simulink model "stab_full_loop"  (R2021a)
settings: Solver=VariableStepAuto  StartTime=0.0  StopTime=5  RelTol=1e-3
values from neighbouring files (symbols this model uses):
  Ahs3 = blkdiag(Ahs3, Ahcs)    [ranger_full_indi_sim.m]
  Ahs7 = blkdiag(Ahs7, Ahcs)    [ranger_full_indi_sim.m]
  Amc = d2c(Amd,'tustin')    [ranger_full_indi_sim.m]
  Asc = d2c(Asd,'tustin')    [ranger_full_indi_sim.m]
  Bhs3 = blkdiag(Bhs3, Bhcs)    [ranger_full_indi_sim.m]
  Bhs7 = blkdiag(Bhs7, Bhcs)    [ranger_full_indi_sim.m]
  Chs3 = blkdiag(Chs3, Chcs)    [ranger_full_indi_sim.m]
  Chs7 = blkdiag(Chs7, Chcs)    [ranger_full_indi_sim.m]
  Dhs3 = blkdiag(Dhs3, Dhcs)    [ranger_full_indi_sim.m]
  Dhs7 = blkdiag(Dhs7, Dhcs)    [ranger_full_indi_sim.m]
  Gs = [-10.67  10.67  0     0     0     0 0 ... (first row only)    [ranger_full_indi_sim.m]
  Gs_inv = pinv(Gs)    [ranger_full_indi_sim.m]
  Gs_thrust = [0 0 0 0 0 0 0 ... (first row only)    [ranger_full_indi_sim.m]
  Kds = [10; 18; 18]    [ranger_full_indi_sim.m]
  Kps = [4.1089; 4.7304; 7.36]    [ranger_full_indi_sim.m]
settings Model: Creator=AutomZ2-RG02B04  LastModifiedBy=AutomZ2-RG02A02
settings SolverCC: AlgebraicLoopSolver=TrustRegion

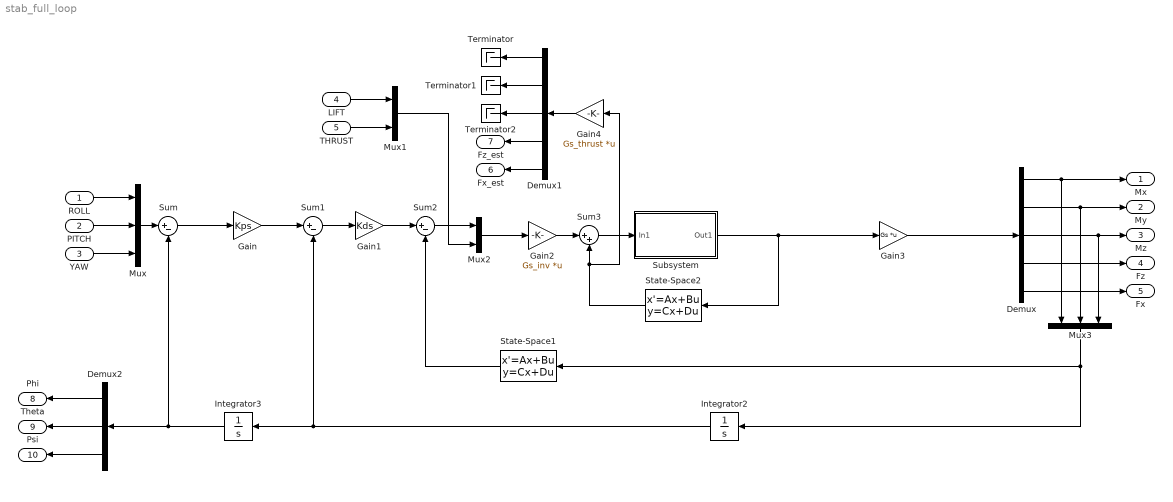
== system stab_full_loop ==
  ROLL : Inport
  PITCH : Inport  Port=2
  YAW : Inport  Port=3
  LIFT : Inport  Port=4
  THRUST : Inport  Port=5
  Demux : Demux  Outputs=5
  Demux1 : Demux  Outputs=5
  Demux2 : Demux  Outputs=3
  Gain : Gain  Gain=Kps
  Gain1 : Gain  Gain=Kds
  Gain2 : Gain  Gain=Gs_inv  Multiplication=Matrix(K*u)
  Gain3 : Gain  Gain=Gs  Multiplication=Matrix(K*u)
  Gain4 : Gain  Gain=Gs_thrust  Multiplication=Matrix(K*u)
  Integrator2 : Integrator
  Integrator3 : Integrator
  Mux : Mux  Inputs=3
  Mux1 : Mux  Inputs=2
  Mux2 : Mux  Inputs=[3 2]
  Mux3 : Mux  Inputs=3
  State-Space1 : StateSpace  A=Ahs3  B=Bhs3  C=Chs3  D=Dhs3  InitialCondition=0
  State-Space2 : StateSpace  A=Ahs7  B=Bhs7  C=Chs7  D=Dhs7  InitialCondition=0
  Subsystem : Subsystem
  Sum : Sum  Inputs=|+-
  Sum1 : Sum  Inputs=|+-
  Sum2 : Sum  Inputs=|+-
  Sum3 : Sum  Inputs=|++
  Terminator : Terminator
  Terminator1 : Terminator
  Terminator2 : Terminator
  Mx : Outport
  My : Outport  Port=2
  Mz : Outport  Port=3
  Fz : Outport  Port=4
  Fx : Outport  Port=5
  Fx_est : Outport  Port=6
  Fz_est : Outport  Port=7
  Phi : Outport  Port=8
  Theta : Outport  Port=9
  Psi : Outport  Port=10
  wires:
  Sum/1 -> Gain/1
  Gain/1 -> Sum1/1
  Sum1/1 -> Gain1/1
  Gain1/1 -> Sum2/1
  Sum2/1 -> Mux2/1
  Gain2/1 -> Sum3/1
  Mux2/1 -> Gain2/1
  Sum3/1 -> Subsystem/1(In1)
  PITCH/1 -> Mux/2
  YAW/1 -> Mux/3
  Mux/1 -> Sum/1
  LIFT/1 -> Mux1/1
  THRUST/1 -> Mux1/2
  Mux1/1 -> Mux2/2
  Demux/1 -> Mux3/1, Mx/1
  Demux/2 -> Mux3/2, My/1
  Demux/3 -> Mz/1, Mux3/3
  Demux/4 -> Fz/1
  Demux/5 -> Fx/1
  Gain4/1 -> Demux1/1
  Demux1/4 -> Fz_est/1
  Demux1/5 -> Fx_est/1
  ROLL/1 -> Mux/1
  Demux1/1 -> Terminator/1
  Demux1/2 -> Terminator1/1
  Demux1/3 -> Terminator2/1
  Gain3/1 -> Demux/1
  Integrator2/1 -> Sum1/2, Integrator3/1
  State-Space2/1 -> Gain4/1, Sum3/2
  State-Space1/1 -> Sum2/2
  Subsystem/1(Out1) -> State-Space2/1, Gain3/1
  Mux3/1 -> State-Space1/1, Integrator2/1
  Integrator3/1 -> Demux2/1, Sum/2
  Demux2/1 -> Phi/1
  Demux2/2 -> Theta/1
  Demux2/3 -> Psi/1

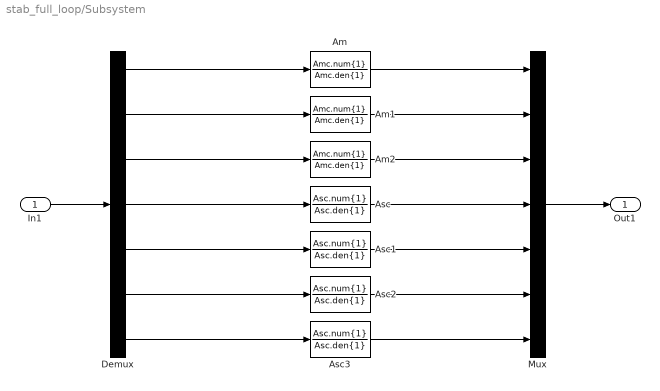
== system stab_full_loop/Subsystem ==
  In1 : Inport
  Am : TransferFcn  Numerator=Amc.num{1}  Denominator=Amc.den{1}
  Am1 : TransferFcn  Numerator=Amc.num{1}  Denominator=Amc.den{1}
  Am2 : TransferFcn  Numerator=Amc.num{1}  Denominator=Amc.den{1}
  Asc{,1..3} (4 alike) : TransferFcn  Numerator=Asc.num{1}  Denominator=Asc.den{1}
  Demux : Demux  Outputs=7
  Mux : Mux  Inputs=7
  Out1 : Outport
  wires:
  Demux/5 -> Asc1/1
  Asc/1 -> Mux/4
  Demux/4 -> Asc/1
  Asc1/1 -> Mux/5
  Asc2/1 -> Mux/6
  Demux/6 -> Asc2/1
  Asc3/1 -> Mux/7
  Demux/7 -> Asc3/1
  In1/1 -> Demux/1
  Mux/1 -> Out1/1
  Demux/1 -> Am/1
  Am/1 -> Mux/1
  Am1/1 -> Mux/2
  Demux/2 -> Am1/1
  Am2/1 -> Mux/3
  Demux/3 -> Am2/1
